simulink model "dc2dc_boost_3"  (Simulink 7.4)
settings: Solver=ode23s  StartTime=0.0  StopTime=.01  MaxStep=.5/Fsw  RelTol=1e-3  AbsTol=1e-3
InitFcn:
  | Fsw=1e6;
libraries: powerlib x13, simulink x3, simulink_extras x1
CloseFcn:
  | rtwprivate ssgencode ModelCloseRequest swps_2
settings Model: Creator=Dick Benson  LastModifiedBy=Dick
settings SolverCC: InitialStep=1e-9  ZeroCrossControl=EnableAll
settings DataIOCC: LimitDataPoints=off  SaveOutput=off  SignalLogging=off  SaveTime=off  SignalLoggingName=sigsOut
settings OptimizationCC: BooleanDataType=off  InitFltsAndDblsToZero=on  OptimizeModelRefInitCode=on  LifeSpan=1
settings DebuggingCC: AlgebraicLoopMsg=none  ArtificialAlgebraicLoopMsg=none  SaveWithParameterizedLinksMsg=none  SignalResolutionControl=TryResolveAllWithWarning  SolverPrmCheckMsg=none  MultiTaskDSMMsg=warning  MultiTaskCondExecSysMsg=none  StrictBusMsg=None
settings RTWCC: SystemTargetFile=ert.tlc  TemplateMakefile=ert_default_tmf  Description=Real-Time Workshop Embedded Coder (no auto configuration)  GenerateReport=on  ProcessScript=ert_make_rtw_hook  IncludeHyperlinkInReport=on  LaunchReport=on  IncludeERTFirstTime=on
settings CodeAppCC: IgnoreCustomStorageClasses=off
settings ERTTargetCC: TargetFcnLib=ansi_tfl_tmw.mat  MultiwordLength=2048  GenerateSampleERTMain=on  GenerateErtSFunction=on  InlinedParameterPlacement=NonHierarchical  ERTCustomFileTemplate=example_file_process.tlc  ConvertIfToSwitch=off

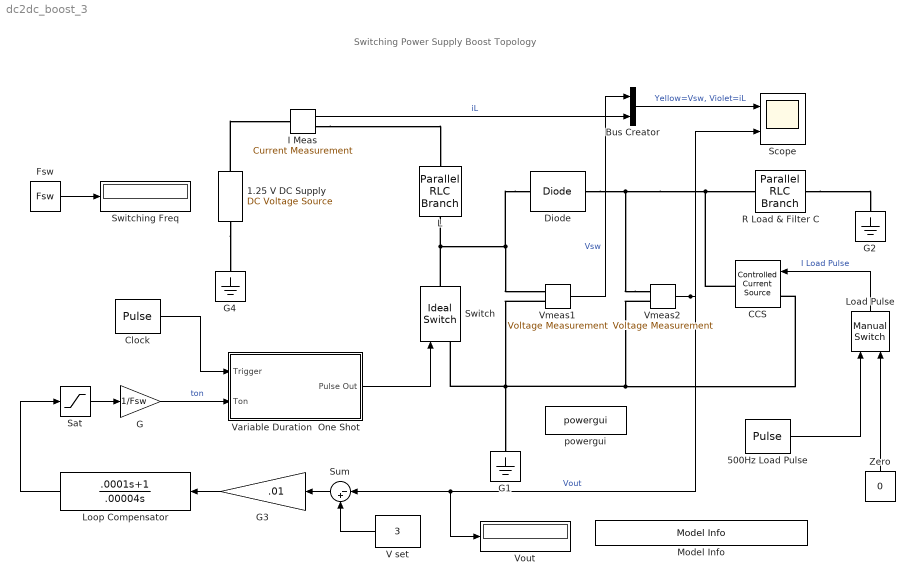
== system dc2dc_boost_3 ==
  note: Switching Power Supply
      | Boost Topology
  1.25 V DC Supply : powerlib/Electrical Sources/DC Voltage Source  Description=source block  DialogController=POWERSYS.PowerSysDialog  SystemSampleTime=-1  Amplitude=1.25  Measurements=None
      settings: AttributesFormatString=\n
  500Hz Load Pulse : DiscretePulseGenerator  PulseType=Time based  Amplitude=-1  Period=1/500  PulseWidth=50  PhaseDelay=1e-6  SampleTime=1
  Bus Creator : BusCreator  Inputs=2
  CCS : powerlib/Electrical Sources/Controlled Current Source  Description=source block  DialogController=POWERSYS.PowerSysDialog  SystemSampleTime=-1  Initialize=off  Source_Type=AC  Amplitude=10  Phase=0  Frequency=0  Measurements=None
      settings: AttributesFormatString=\n
  Clock : DiscretePulseGenerator  PulseType=Time based  Amplitude=1  Period=1/Fsw  PulseWidth=50  PhaseDelay=1e-6  SampleTime=1
  Diode : powerlib/Power Electronics/Diode  DialogController=POWERSYS.PowerSysDialog  SystemSampleTime=-1  Ron=.025  Lon=0  Vf=.5  IC=0  UseSnubber=off  Rs=inf  Cs=0  Measurements=off
  Fsw : Constant  Value=Fsw  OutDataType=sfix(16)  OutScaling=2^0
  G : Gain  Gain=1/Fsw  ParameterDataType=sfix(16)  ParameterScaling=2^0  OutDataType=sfix(16)  OutScaling=2^0  SaturateOnIntegerOverflow=on  OutDataTypeStr=Inherit: Same as input  ParamDataTypeStr=Inherit: Same as input
  G1 : powerlib/Elements/Ground  DialogController=POWERSYS.PowerSysDialog  PhysicalDomain=powersysdomain  SubClassName=unknown  LeftPortType=p1  RightPortType=p1  LConnTagsString=a
  G2 : powerlib/Elements/Ground  DialogController=POWERSYS.PowerSysDialog  PhysicalDomain=powersysdomain  SubClassName=unknown  LeftPortType=p1  RightPortType=p1  LConnTagsString=a
  G3 : Gain  Gain=.01  ParameterDataType=sfix(16)  ParameterScaling=2^0  OutDataType=sfix(16)  OutScaling=2^0  SaturateOnIntegerOverflow=on  OutDataTypeStr=Inherit: Same as input  ParamDataTypeStr=Inherit: Same as input
  G4 : powerlib/Elements/Ground  DialogController=POWERSYS.PowerSysDialog  PhysicalDomain=powersysdomain  SubClassName=unknown  LeftPortType=p1  RightPortType=p1  LConnTagsString=a
  I Meas : powerlib/Measurements/Current Measurement  DialogController=POWERSYS.PowerSysDialog  SystemSampleTime=-1  PhasorSimulation=off  OutputType=Complex  PSBequivalent=0
  L : powerlib/Elements/Parallel RLC Branch  DialogController=POWERSYS.PowerSysDialog  PhysicalDomain=powersysdomain  SubClassName=unknown  LeftPortType=p1  RightPortType=p1  LConnTagsString=a  RConnTagsString=__new0  BranchType=RL  Resistance=1000  Inductance=1e-6  SetiL0=off  InitialCurrent=0  Capacitance=1.0  Setx0=off  InitialVoltage=0  Measurements=None
  Load Pulse : simulink/Signal Routing/Manual Switch  SystemSampleTime=-1  sw=1  action=0  varsize=off
  Loop Compensator : TransferFcn  Numerator=[.0001 1]  Denominator=[.00004 0]
  Model Info : simulink/Model-Wide Utilities/Model Info  SystemSampleTime=-1  InitialBlockCM=None  BlockCM=None  Frame=on  DisplayStringWithTags=Copywrite 2010 The MathWorks, Inc.  HorizontalTextAlignment=Center  LeftAlignmentValue=0.5  SourceBlockDiagram=dc2dc_boost_3  TagMaxNumber=20
  R Load & Filter C : powerlib/Elements/Parallel RLC Branch  DialogController=POWERSYS.PowerSysDialog  PhysicalDomain=powersysdomain  SubClassName=unknown  LeftPortType=p1  RightPortType=p1  LConnTagsString=a  RConnTagsString=__new0  BranchType=RC  Resistance=3  Inductance=1.0  SetiL0=off  InitialCurrent=0  Capacitance=120e-6  Setx0=off  InitialVoltage=0  Measurements=None
  Sat : Saturate  UpperLimit=0.8  LowerLimit=.01
  Scope : Scope  NumInputPorts=2
      settings: TimeRange=0.01  YMin=0~0  YMax=10~3.5  SaveName=ScopeData2
  Sum : Sum  Inputs=|-+  OutDataType=sfix(16)  OutScaling=2^0  SaturateOnIntegerOverflow=on  InputSameDT=on  OutDataTypeStr=Inherit: Same as first input
  Switch : powerlib/Power Electronics/Ideal Switch  DialogController=POWERSYS.PowerSysDialog  SystemSampleTime=-1  Ron=0.02  Lon=0  IC=0  Rs=0  Cs=0  Measurements=off
      settings: AttributesFormatString=\n
  Switching Freq : Display
  "V set " : Constant  Value=3  OutDataType=sfix(16)  OutScaling=2^0
  Variable Duration  One Shot : Subsystem
  Vmeas1 : powerlib/Measurements/Voltage Measurement  Tag=PoWeRsYsTeMmEaSuReMeNt  DialogController=POWERSYS.PowerSysDialog  SystemSampleTime=-1  PhasorSimulation=off  OutputType=Magnitude  PSBequivalent=0
  Vmeas2 : powerlib/Measurements/Voltage Measurement  Tag=PoWeRsYsTeMmEaSuReMeNt  DialogController=POWERSYS.PowerSysDialog  SystemSampleTime=-1  PhasorSimulation=off  OutputType=Magnitude  PSBequivalent=0
  Vout : Display
      settings: Decimation=20
  Zero : Constant  Value=0  OutDataType=sfix(16)  OutScaling=2^0
  powergui : powerlib/powergui  SystemSampleTime=-1  SimulationMode=Continuous  SampleTime=0  frequency=60  SPID=off  DisableSnubberDevices=off  DisableRonSwitches=off  DisableVfSwitches=off  SwTol=0  Interpol=off  frequencyindice=0  echomessages=off  HookPort=off  DisplayEquations=off  FunctionMessages=off  EnableUseOfTLC=off  x0status=blocks  RestoreLinks=warning  Frange=[0:2:500]  Ylog=off  Xlog=on  ShowGrid=off  save=off  variable=ZData  ZoomFFT=on  StartTime=0.0  cycles=1  DisplayStyle=1  fundamental=60  FreqAxis=off  MaxFrequency=1000  frequencyindicesteady=1  RmsSteady=1  display=off  Ts=0  methode=off
  wires:
  Clock/1 -> Variable Duration  One Shot/1(Trigger)
  Sum/1 -> G3/1
  "V set "/1 -> Sum/2
  G/1 -> Variable Duration  One Shot/2(Ton)  "ton"
  500Hz Load Pulse/1 -> Load Pulse/1
  Zero/1 -> Load Pulse/2
  G3/1 -> Loop Compensator/1
  Vmeas2/1 -> Sum/1, Vout/1, Scope/2  "Vout"
  Load Pulse/1 -> CCS/1  "I Load Pulse"
  Loop Compensator/1 -> Sat/1
  Variable Duration  One Shot/1(Pulse Out) -> Switch/1
  Sat/1 -> G/1
  Fsw/1 -> Switching Freq/1
  Bus Creator/1 -> Scope/1  "Yellow=Vsw, Violet=iL"
  Vmeas1/1 -> Bus Creator/1  "Vsw"
  I Meas/1 -> Bus Creator/2  "iL"
  connections:
  R Load & Filter C/RConn1 -- G2/LConn1
  Diode/LConn1 -- Switch/RConn1 -- L/RConn1 -- Vmeas1/LConn1
  Vmeas2/LConn1 -- Diode/RConn1 -- R Load & Filter C/LConn1 -- CCS/RConn1
  Vmeas2/LConn2 -- Vmeas1/LConn2 -- Switch/LConn1 -- G1/LConn1 -- CCS/LConn1
  I Meas/RConn1 -- L/LConn1
  1.25 V DC Supply/LConn1 -- G4/LConn1
  1.25 V DC Supply/RConn1 -- I Meas/LConn1

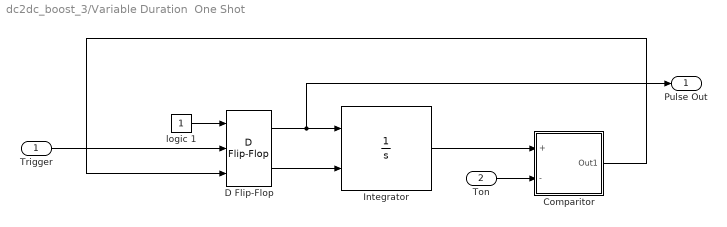
== system dc2dc_boost_3/Variable Duration  One Shot ==
  Trigger : Inport  OutDataType=sfix(16)  OutScaling=2^0
  Ton : Inport  Port=2  OutDataType=sfix(16)  OutScaling=2^0
  Comparitor : Subsystem
  D Flip-Flop : simulink_extras/Flip Flops/D Flip-Flop  SystemSampleTime=-1
  Integrator : Integrator  ExternalReset=level
  logic 1 : Constant  OutDataType=sfix(16)  OutScaling=2^0
  Pulse Out : Outport  OutDataType=sfix(16)  OutScaling=2^0
  wires:
  D Flip-Flop/2 -> Integrator/2
  logic 1/1 -> D Flip-Flop/1
  Integrator/1 -> Comparitor/1(+)
  D Flip-Flop/1 -> Integrator/1, Pulse Out/1
  Trigger/1 -> D Flip-Flop/2
  Ton/1 -> Comparitor/2(-)
  Comparitor/1(Out1) -> D Flip-Flop/3

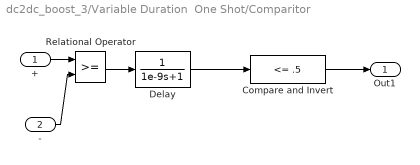
== system dc2dc_boost_3/Variable Duration  One Shot/Comparitor ==
  + : Inport  OutDataType=sfix(16)  OutScaling=2^0
  - : Inport  Port=2  OutDataType=sfix(16)  OutScaling=2^0
  "Compare and Invert " : simulink/Logic and Bit Operations/Compare To Constant  SystemSampleTime=-1  relop=<=  const=.5  LogicOutDataTypeMode=uint8  ZeroCross=off
  Delay : TransferFcn  Denominator=[1e-9 1]
  Relational Operator : RelationalOperator  InputSameDT=on
  Out1 : Outport  OutDataType=sfix(16)  OutScaling=2^0
  wires:
  Relational Operator/1 -> Delay/1
  +/1 -> Relational Operator/1
  Delay/1 -> "Compare and Invert "/1
  -/1 -> Relational Operator/2
  "Compare and Invert "/1 -> Out1/1
